simulink model "Oving1Oppg1"  (R2020b)
settings: Solver=VariableStepAuto  StartTime=0.0  StopTime=100.0  RelTol=1e-3
values from neighbouring files (symbols this model uses):
  A = 1    [Oving1Oppg1.mat]
  k = 1    [Oving1Oppg1.mat]
  k_p = 1    [Oving1Oppg1.mat]
  r = 1    [Oving1Oppg1.mat]
  w = 1    [Oving1Oppg1.mat]
undefined symbols (not defined in the file or in its folder): x_0
settings Model: Creator=crezl  LastModifiedBy=crezl

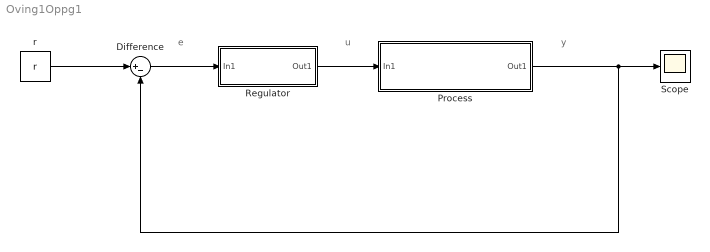
== system Oving1Oppg1 ==
  note: e
  note: u
  note: y
  Difference : Sum  Inputs=|+-
  Process : Subsystem
  Regulator : Subsystem
  Scope : Scope
  r : Constant  Value=r
  wires:
  r/1 -> Difference/1
  Difference/1 -> Regulator/1(In1)
  Process/1(Out1) -> Difference/2, Scope/1
  Regulator/1(Out1) -> Process/1(In1)

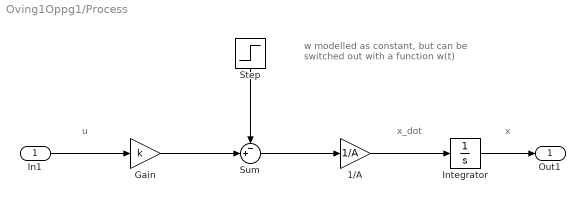
== system Oving1Oppg1/Process ==
  note: w modelled as constant, but can be
      | switched out with a function w(t)
  note: u
  note: x
  note: x_dot
  In1 : Inport
  1/A : Gain  Gain=1/A
  Gain : Gain  Gain=k
  Integrator : Integrator  InitialCondition=x_0
  Step : Step  Time=10  After=w  SampleTime=0
  Sum : Sum  Inputs=-+|
  Out1 : Outport
  wires:
  Sum/1 -> 1/A/1
  1/A/1 -> Integrator/1
  Step/1 -> Sum/1
  Integrator/1 -> Out1/1
  In1/1 -> Gain/1
  Gain/1 -> Sum/2

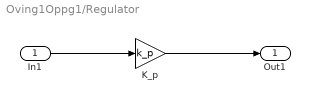
== system Oving1Oppg1/Regulator ==
  In1 : Inport
  K_p : Gain  Gain=k_p
  Out1 : Outport
  wires:
  K_p/1 -> Out1/1
  In1/1 -> K_p/1
